simulink model "MOAB"  (R2020a)
settings: Solver=ode23t  StartTime=0.0  StopTime=Inf  RelTol=1e-3  AbsTol=1e-3
undefined symbols (not defined in the file or in its folder): ball_mass, ball_radius, ball_shell, DEFAULT_BALL_NOISE, DEFAULT_GRAVITY, DEFAULT_PLATE_NOISE, DEFAULT_SIMULATION_RATE, DEFAULT_VEL_NOISE, MAX_ITER, noise_mean, noise_variance, obstacle_radius, plate_pos_z0, plate_radius, smiData, target_pos_x, target_pos_y, tilt_acc, tilt_limit, tilt_max_vel, tilt_x0, tilt_y0, TIME_DELTA, X, Y, Z, z_offset
libraries: sm_lib x119, nesl_utility x21, simulink x1
(part 4 of 4)

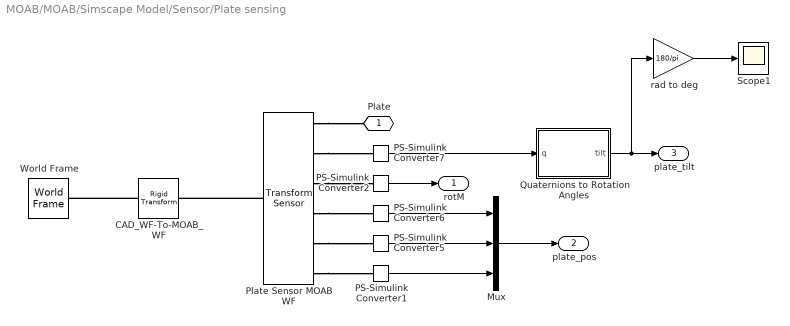
== system MOAB/MOAB/Simscape Model/Sensor/Plate sensing ==
  CAD_WF-To-MOAB_WF : sm_lib/Frames and Transforms/Rigid Transform  TranslationMethod=StandardAxis  TranslationStandardOffset=z_offset  TranslationLengthUnit=m  TranslationStandardAxis=+Z  TranslationCartesianOffset=[0 0 0]  TranslationROffset=0  TranslationROffsetUnits=m  TranslationZOffset=0  TranslationZOffsetUnits=m  TranslationThetaOffset=0  TranslationThetaOffsetUnits=deg  RotationMethod=None  RotationAngleUnits=deg  RotationStandardAxis=+Z  RotationAngle=0.0  RotationArbitraryAxis=[0 0 1]  FollAlignAxisA=+X  BaseAlignAxisA=+Y  FollAlignAxisB=+Y  BaseAlignAxisB=+Z  RotationSequenceAxes=FollowerAxes  RotationSequence=XYX  RotationSequenceAngles=[0 0 0]  RotationSequenceAnglesUnits=deg  RotationMatrix=[1 0 0; 0 1 0; 0 0 1]
  Mux : Mux  Inputs=3
  PS-Simulink Converter1 : nesl_utility/PS-Simulink Converter  PhysicalDomain=network_engine_domain  SubClassName=ps_output  LeftPortType=input  RightPortType=output  PseudoPeriodic=off  Frequencies=[]  Unit=m  AffineConversion=off
  PS-Simulink Converter2 : nesl_utility/PS-Simulink Converter  PhysicalDomain=network_engine_domain  SubClassName=ps_output  LeftPortType=input  RightPortType=output  PseudoPeriodic=off  Frequencies=[]  Unit=inherit  AffineConversion=off
  PS-Simulink Converter5 : nesl_utility/PS-Simulink Converter  PhysicalDomain=network_engine_domain  SubClassName=ps_output  LeftPortType=input  RightPortType=output  PseudoPeriodic=off  Frequencies=[]  Unit=m  AffineConversion=off
  PS-Simulink Converter6 : nesl_utility/PS-Simulink Converter  PhysicalDomain=network_engine_domain  SubClassName=ps_output  LeftPortType=input  RightPortType=output  PseudoPeriodic=off  Frequencies=[]  Unit=m  AffineConversion=off
  PS-Simulink Converter7 : nesl_utility/PS-Simulink Converter  PhysicalDomain=network_engine_domain  SubClassName=ps_output  LeftPortType=input  RightPortType=output  PseudoPeriodic=off  Frequencies=[]  Unit=inherit  AffineConversion=off
  Plate Sensor MOAB WF : sm_lib/Frames and Transforms/Transform Sensor  MeasurementFrame=World  SenseAngle=off  SenseAxis=off  SenseAngle1=off  SenseAngle2=off  SenseAngle3=off  SenseQ=on  SenseR=on  SenseOmegaX=off  SenseOmegaY=off  SenseOmegaZ=off  SenseOmega1=off  SenseOmega2=off  SenseOmega3=off  SenseQDot=off  SenseRDot=off  SenseAlphaX=off  SenseAlphaY=off  SenseAlphaZ=off  SenseAlpha1=off  SenseAlpha2=off  SenseAlpha3=off  SenseQDDot=off  SenseRDDot=off  SenseX=on  SenseY=on  SenseZ=on  SenseRad=off  SenseAzim=off  SenseDist=off  SenseInc=off  SenseXDot=off  SenseYDot=off  SenseZDot=off  SenseRadDot=off  SenseAzimDot=off  SenseDistDot=off  SenseIncDot=off  SenseXDDot=off  SenseYDDot=off  SenseZDDot=off  SenseRadDDot=off  SenseAzimDDot=off  SenseDistDDot=off  SenseIncDDot=off
  Quaternions to Rotation Angles : MATLAB Function  TreatAsAtomicUnit=on
  Scope1 : Scope
  World Frame : sm_lib/Frames and Transforms/World Frame
  rad to deg : Gain  Gain=180/pi
  Plate : PMIOPort  Side=Left
  rotM : Outport
  plate_pos : Outport  Port=2
  plate_tilt : Outport  Port=3
  wires:
  PS-Simulink Converter2/1 -> rotM/1
  PS-Simulink Converter7/1 -> Quaternions to Rotation Angles/1(q)
  PS-Simulink Converter5/1 -> Mux/2
  Mux/1 -> plate_pos/1
  PS-Simulink Converter6/1 -> Mux/1
  PS-Simulink Converter1/1 -> Mux/3
  Quaternions to Rotation Angles/1(tilt) -> plate_tilt/1, rad to deg/1
  rad to deg/1 -> Scope1/1
  connections:
  Plate Sensor MOAB WF/RConn6 -- PS-Simulink Converter1/LConn1
  Plate Sensor MOAB WF/RConn5 -- PS-Simulink Converter5/LConn1
  Plate Sensor MOAB WF/RConn1 -- Plate/RConn1
  Plate Sensor MOAB WF/RConn2 -- PS-Simulink Converter7/LConn1
  Plate Sensor MOAB WF/RConn4 -- PS-Simulink Converter6/LConn1
  Plate Sensor MOAB WF/LConn1 -- CAD_WF-To-MOAB_WF/RConn1
  CAD_WF-To-MOAB_WF/LConn1 -- World Frame/RConn1
  Plate Sensor MOAB WF/RConn3 -- PS-Simulink Converter2/LConn1

== matlab function MOAB/Inverse Kinematics/MATLAB Function ==
  data: plate_height input; alpha output; tilt_x input; tilt_y input; plate_noise input
function alpha = actionsToServoAngles(plate_height, tilt_x, tilt_y, plate_noise)

% add plate noise to x and y tilt
tilt_x = tilt_x + plate_noise;
tilt_y = tilt_y + plate_noise;

% calculate servo joint angles (deg)
[a1,a2,a3] = runMixer(plate_height, tilt_x, tilt_y);

alpha = [a1 a2 a3]';

== matlab function MOAB/Simscape Model/Sensor/Plate sensing/Quaternions to Rotation Angles ==
  data: q input; tilt output
function tilt = quat2tilt(q)
% Quaternion to Euler angle transformation
% Source: https://en.wikipedia.org/wiki/Conversion_between_quaternions_and_Euler_angles

% unpack quaternion
q0 = q(1);
q1 = q(2);
q2 = q(3);
q3 = q(4);

tilt = zeros(3,1);

% tilt about X axis (tilt_y or roll)
tilt(1) = atan2(2*(q0*q1+q2*q3),1-2*(q1^2+q2^2));

% tilt about Y axis (tilt_x or pitch)
tilt(2) = asin(2*(q0*q2-q3*q1));

% tilt about Z axis (yaw)
tilt(3) = atan2(2*(q0*q3+q2*q1),1-2*(q2^2+q3^2));

== matlab function MOAB/Simscape Model/Sensor/Obstacle Sensing/MATLAB Function ==
  data: ball_x input; angle output; ball_y input; vel_x input; vel_y input; point_x input; point_y input
function angle = fcn(ball_x, ball_y, vel_x, vel_y, point_x, point_y)

% vector to point
dx = point_x - ball_x;
dy = point_y - ball_y;

% vectors and lengths
u = [dx, dy, 0.0]./norm([dx, dy, 0.0]);
v = [vel_x, vel_y, 0.0]./norm([vel_x, vel_y, 0.0]);
ul = length(u);
vl = length(v);

% no velocity? already on the target?
angle = 0.0;
if (ul ~= 0.0) && (vl ~= 0.0)
    % angle between vectors
    uv_dot = dot(u,v);

    % signed angle
    x = u(1);
    y = u(2);
    angle = atan2(dot([-y, x, 0.0], v), uv_dot);
    if isnan(angle)
        angle = 0.0;
    end
end

== matlab function MOAB/Controller/Bonsai/Bonsai ==
  data: state input; action output; halted input; reset output
function [action, reset]= fcn(state, halted)
end
